simulink model "empc_yalmip_buck_scale_sl"  (R2024b)
settings: Solver=FixedStepAuto  StartTime=0.0  StopTime=N*T_sw  FixedStep=dt_sim  MaxStep=T_sw/70  RelTol=1e-4
values from neighbouring files (symbols this model uses):
  f_sw = 500e3    (= 500000)    [analog_design_estimator.m]    (also in empc_yalmip_buck_scale_mat.m)
  io = (I_max - 5/RL)    [empc_yalmip_buck_scale_mat.m]
  ks_d = 1    [empc_yalmip_buck_scale_mat.m]
  ks_i_L = 5    [empc_yalmip_buck_scale_mat.m]
  ks_io = 10    [empc_yalmip_buck_scale_mat.m]
  ks_v_C = 1    [empc_yalmip_buck_scale_mat.m]
  ks_v_in = 1    [empc_yalmip_buck_scale_mat.m]
  N_io_end = 1100    [empc_yalmip_buck_scale_mat.m]
  N_io_start = 1000    [empc_yalmip_buck_scale_mat.m]
  N_v_in_end = 1300    [empc_yalmip_buck_scale_mat.m]
  N_v_in_start = 1200    [empc_yalmip_buck_scale_mat.m]
  Rc_nominal = 50e-3    (= 0.05)    [empc_yalmip_buck_scale_mat.m]
  RL_nominal = mean(RL_range)    [analog_design_estimator.m]    (also in empc_yalmip_buck_scale_mat.m)
  T_sw = 1/f_sw    (= 2e-06)    [analog_design_estimator.m]    (also in empc_yalmip_buck_scale_mat.m)
  V_in = V_in_nominal    (= 50)    [analog_design_estimator.m]    (also in empc_yalmip_buck_scale_mat.m)
  v_in = 10    [empc_yalmip_buck_scale_mat.m]
  x0 = [0, 0]'    [empc_yalmip_buck_scale_mat.m]
libraries: simulink x2, cstblocks x1
settings Model: Creator=Lorenzo  LastModifiedBy=simon
settings SolverCC: ZeroCrossAlgorithm=Adaptive  AlgebraicLoopSolver=TrustRegion
settings DebuggingCC: AlgebraicLoopMsg=none  IgnoredZcDiagnostic=none  UnconnectedInputMsg=warning  UnconnectedOutputMsg=warning  UnconnectedLineMsg=warning
settings ModelReferenceCC: EnableRefExpFcnMdlSchedulingChecks=on
settings RTWCC: GPUComputeCapability=3.5  DLArmComputeVersion=19.05

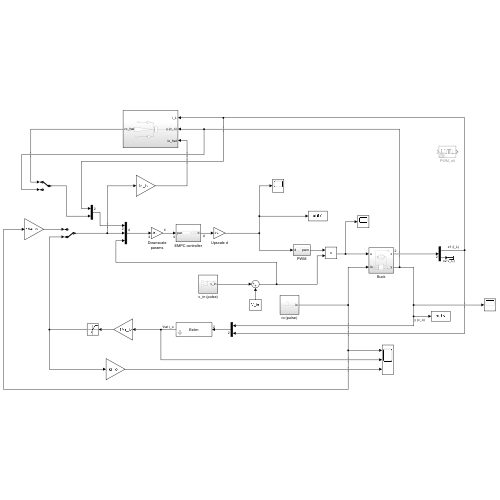
[thumbnail: Simulink's stored preview of the top-level diagram]
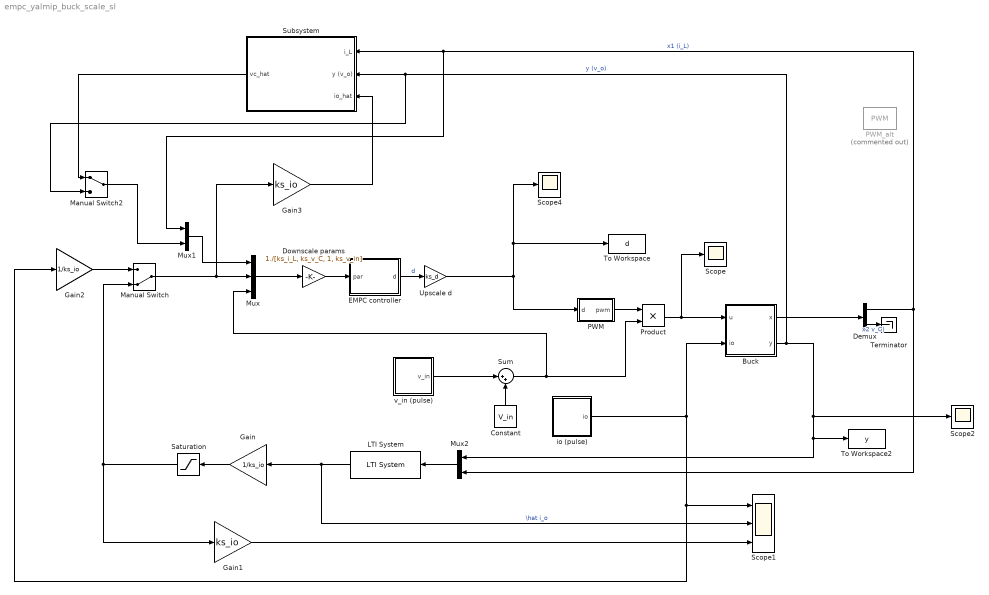
== system empc_yalmip_buck_scale_sl ==
  Buck : Subsystem
  Constant : Constant  Value=V_in
  Demux : Demux  Outputs=2
  Downscale params : Gain  Gain=1./[ks_i_L, ks_v_C, 1, ks_v_in]
  EMPC controller : Subsystem
  Gain : Gain  Gain=1/ks_io
  Gain1 : Gain  Gain=ks_io
  Gain2 : Gain  Gain=1/ks_io
  Gain3 : Gain  Gain=ks_io
  LTI System : cstblocks/LTI System  sys=Estim  IC=[]  PadeOrder=0
  Manual Switch : ManualSwitch  CurrentSetting=0
  Manual Switch2 : ManualSwitch
  Mux : Mux  Inputs=3
  Mux1 : Mux  Inputs=2
  Mux2 : Mux  Inputs=2
  PWM : Subsystem
  PWM_alt : simulink/Discontinuities/PWM  Commented=on  DisableCoverage=on  Period=T_sw  InitialDelay=0  DisallowZeroDutyCycle=off  RunAtFixedTimeIntervals=off  SampleTime=0.1
  Product : Product
  Saturation : Saturate  UpperLimit=5  LowerLimit=0
  Scope : Scope
  Scope1 : Scope  NumInputPorts=3
  Scope2 : Scope
  Scope4 : Scope
  Subsystem : Subsystem
  Sum : Sum  Inputs=|++
  Terminator : Terminator
  To Workspace : ToWorkspace  VariableName=d  SaveFormat=Timeseries  SampleTime=-1
  To Workspace2 : ToWorkspace  VariableName=y  SaveFormat=Timeseries  SampleTime=-1
  Upscale d : Gain  Gain=ks_d
  io (pulse) : Subsystem
  v_in (pulse) : Subsystem
  wires:
  EMPC controller/1(d) -> Upscale d/1  "d"
  Buck/2(y) -> Mux2/1, To Workspace2/1, Scope2/1, Manual Switch2/2, Subsystem/2(y (v_o))  "y (v_o)"
  Demux/1 -> Mux1/1, Subsystem/1(i_L), Mux2/2  "x1 (i_L)"
  Constant/1 -> Sum/2
  Product/1 -> Buck/1(u), Scope/1
  Sum/1 -> Mux/3, Product/2
  io (pulse)/1(io) -> Gain2/1, Scope1/1, Buck/2(io)
  Buck/1(x) -> Demux/1
  PWM/1(pwm) -> Product/1
  Mux/1 -> Downscale params/1
  Downscale params/1 -> EMPC controller/1(par)
  LTI System/1 -> Scope1/2, Gain/1  "\\hat i_o"
  Mux2/1 -> LTI System/1
  Gain/1 -> Saturation/1
  Manual Switch/1 -> Mux/2, Gain3/1
  Upscale d/1 -> To Workspace/1, Scope4/1, PWM/1(d)
  Saturation/1 -> Manual Switch/2, Gain1/1
  Gain1/1 -> Scope1/3
  v_in (pulse)/1(v_in) -> Sum/1
  Gain2/1 -> Manual Switch/1
  Gain3/1 -> Subsystem/3(io_hat)
  Mux1/1 -> Mux/1
  Manual Switch2/1 -> Mux1/2
  Subsystem/1(vc_hat) -> Manual Switch2/1
  Demux/2 -> Terminator/1  "x2 v_C)"

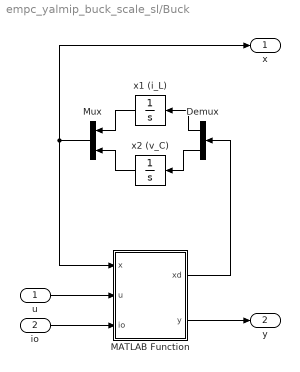
== system empc_yalmip_buck_scale_sl/Buck ==
  u : Inport
  io : Inport  Port=2
  Demux : Demux  Outputs=2
  MATLAB Function : MATLAB Function  TreatAsAtomicUnit=on
  Mux : Mux  Inputs=2
  x1 (i_L) : Integrator  InitialCondition=x0(1)  LimitOutput=on  LowerSaturationLimit=0
  x2 (v_C) : Integrator  InitialCondition=x0(2)
  x : Outport
  y : Outport  Port=2
  wires:
  u/1 -> MATLAB Function/2(u)
  io/1 -> MATLAB Function/3(io)
  MATLAB Function/2(y) -> y/1
  MATLAB Function/1(xd) -> Demux/1
  Demux/1 -> x1 (i_L)/1
  Demux/2 -> x2 (v_C)/1
  x1 (i_L)/1 -> Mux/1
  x2 (v_C)/1 -> Mux/2
  Mux/1 -> x/1, MATLAB Function/1(x)

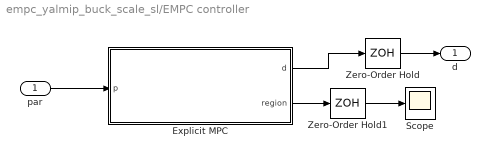
== system empc_yalmip_buck_scale_sl/EMPC controller ==
  par : Inport
  Explicit MPC : MATLAB Function  TreatAsAtomicUnit=on
  Scope : Scope
  Zero-Order Hold : ZeroOrderHold  SampleTime=T_sw
  Zero-Order Hold1 : ZeroOrderHold  SampleTime=T_sw
  d : Outport
  wires:
  Explicit MPC/1(d) -> Zero-Order Hold/1
  par/1 -> Explicit MPC/1(p)
  Zero-Order Hold/1 -> d/1
  Explicit MPC/2(region) -> Zero-Order Hold1/1
  Zero-Order Hold1/1 -> Scope/1

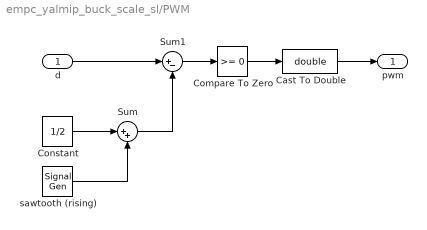
== system empc_yalmip_buck_scale_sl/PWM ==
  d : Inport
  Cast To Double : DataTypeConversion  OutMin=0  OutMax=1  OutDataTypeStr=double  RndMeth=Round  SaturateOnIntegerOverflow=off
  Compare To Zero : simulink/Logic and Bit Operations/Compare To Zero  relop=>=  OutDataTypeStr=boolean
  Constant : Constant  Value=1/2
  Sum : Sum  Inputs=|++
  Sum1 : Sum  Inputs=|+-
  sawtooth (rising) : SignalGenerator  WaveForm=sawtooth  Amplitude=-1/2  Frequency=f_sw
  pwm : Outport
  wires:
  Constant/1 -> Sum/1
  sawtooth (rising)/1 -> Sum/2
  Cast To Double/1 -> pwm/1
  Compare To Zero/1 -> Cast To Double/1
  Sum/1 -> Sum1/2
  Sum1/1 -> Compare To Zero/1
  d/1 -> Sum1/1

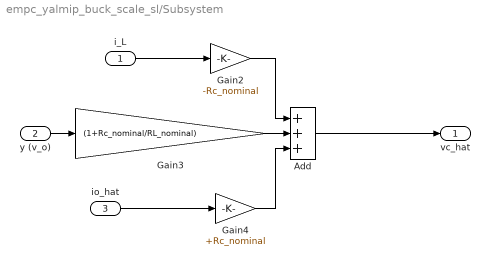
== system empc_yalmip_buck_scale_sl/Subsystem ==
  i_L : Inport
  y (v_o) : Inport  Port=2
  io_hat : Inport  Port=3
  Add : Sum  Inputs=+++
  Gain2 : Gain  Gain=-Rc_nominal
  Gain3 : Gain  Gain=(1+Rc_nominal/RL_nominal)
  Gain4 : Gain  Gain=+Rc_nominal
  vc_hat : Outport
  wires:
  y (v_o)/1 -> Gain3/1
  Add/1 -> vc_hat/1
  Gain4/1 -> Add/3
  io_hat/1 -> Gain4/1
  i_L/1 -> Gain2/1
  Gain3/1 -> Add/2
  Gain2/1 -> Add/1

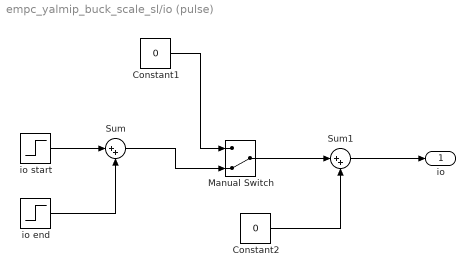
== system empc_yalmip_buck_scale_sl/io (pulse) ==
  Constant1 : Constant  Value=0
  Constant2 : Constant  Value=0
  Manual Switch : ManualSwitch  CurrentSetting=0
  Sum : Sum  Inputs=|++
  Sum1 : Sum  Inputs=|++
  io end : Step  Time=N_io_end*T_sw  After=-0.8*io  SampleTime=0
  io start : Step  Time=N_io_start*T_sw  After=io  SampleTime=0
  io : Outport
  wires:
  Sum1/1 -> io/1
  Manual Switch/1 -> Sum1/1
  io start/1 -> Sum/1
  io end/1 -> Sum/2
  Sum/1 -> Manual Switch/2
  Constant1/1 -> Manual Switch/1
  Constant2/1 -> Sum1/2

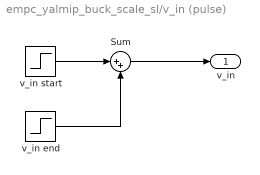
== system empc_yalmip_buck_scale_sl/v_in (pulse) ==
  Sum : Sum  Inputs=|++
  v_in end : Step  Time=N_v_in_end*T_sw  After=-v_in  SampleTime=0
  v_in start : Step  Time=N_v_in_start*T_sw  After=v_in  SampleTime=0
  v_in : Outport
  wires:
  Sum/1 -> v_in/1
  v_in start/1 -> Sum/1
  v_in end/1 -> Sum/2

== matlab function empc_yalmip_buck_scale_sl/EMPC controller/Explicit MPC ==
  data: p input size=4; d output size=1; data parameter; region output
function [d,region] = empc_controller(p, data)

d = -1;

ks_d = data.ks_d;

n_reg = data.n_reg;
H = data.H;
F = data.F;
g = data.g;
ni = data.ni;

a_opt = data.a_opt;
b_opt = data.b_opt;

sep_fun = @(x) a_opt*x + b_opt;

%p = [x; io; v_in]; % Param value

region = 0;
ph = [p; -1];
for i=1:1:n_reg
	if all( H( (ni(i)+1):1:(ni(i+1)) , : )*ph <= 1e-08 ) % Check non-saturated region
		d = F(i,:)*p + g(i); % Compute affine function
		region = i;
		break
	end
end

if region == 0 % p is in a saturated region
	sep_val = sep_fun(p);
	if sep_val > 0
		d = 1/ks_d;
	else
		d = 0/ks_d;
	end
end

end

== matlab function empc_yalmip_buck_scale_sl/Buck/MATLAB Function ==
  data: x input size=2; xd output size=2; u input size=1; y output size=1; io input size=1; data parameter
function [xd, y] = buck_ct(x,u,io,data)

A = data.A;
B1 = data.B1;
B2 = data.B2;
C = data.C;
D1 = data.D1;

xd = A*x + B1*io + B2*u;
y = C*x + D1*io;

end
